simulink model "DeathOrGlory"  (R2017b)
settings: Solver=ode3  StartTime=0.0  StopTime=inf  FixedStep=0.0005  RelTol=1e-3
values from neighbouring files (symbols this model uses):
  fs = 1000    [Acquisizione_segnale_per_SVM_prova.m]    (also in training.m; warmup.m)
  interval = 192    [warmup.m]
  null_sum_finger = null_base_finger(:,1)+null_base_finger(:,2)    [matrix_h_hand_config.m]
  null_sum_thumb = null_base_thumb(:,1)+null_base_thumb(:,2)    [matrix_h_hand_config.m]
  num_act = 30    [KinematicData.m]
  pseudo_inv_h_finger = pinv(h_finger)    [matrix_h_hand_config.m]
  pseudo_inv_h_thumb = pinv(h_thumb)    [matrix_h_hand_config.m]
  pseudo_inv_h_wrist = pinv(h_wrist)    [matrix_h_hand_config.m]
  pseudo_inv_trasp_h_finger = pinv(transp(h_finger))    [matrix_h_hand_config.m]
  pseudo_inv_trasp_h_thumb = pinv(transp(h_thumb))    [matrix_h_hand_config.m]
  pseudo_inv_trasp_h_wrist = pinv(transp(h_wrist))    [matrix_h_hand_config.m]
  sM = mean(train(:,1:end-1))    [SVM_crossValidation.m]    (also in training.m; warmup.m = 0)
  sS = std(train(:,1:end-1))    [SVM_crossValidation.m]    (also in training.m; warmup.m = 0)
  Temg = 0.0005    [START_parametri_simulink.mat]    (also in matrix_h_hand_config.m)
  Ts = 0.05    [KinematicData.m]    (also in START_parametri_simulink.mat)
  w = 20    [Acquisizione_segnale_per_SVM_prova.m]    (also in warmup.m)
libraries: simulink x28, dspindex x15, dspfdesign x2, simulink_need_slupdate x2, dspmlti4 x1, dspstat3 x1, dspsrcs4 x1, simulink_extras x1
(part 2 of 2)

== system DeathOrGlory/UB Hand system1/SEND REFERENCES/dyna_send/Subsystem7 ==
  In1 : Inport
  Add : Sum  Inputs=+-
  Interval Test : simulink/Logic and Bit Operations/Interval Test  IntervalClosedRight=on  uplimit=0.1  IntervalClosedLeft=on  lowlimit=-0.1  OutDataTypeStr=boolean
  Logical Operator : Logic  Operator=NOT  AllPortsSameDT=off  OutDataTypeStr=boolean
  Unit Delay : UnitDelay  InitialCondition=zeros(30,1)  SampleTime=-1
  tag scope: changes_punch=global
  wires:
  Unit Delay/1 -> Add/2
  Add/1 -> Interval Test/1
  Interval Test/1 -> Logical Operator/1
  In1/1 -> Unit Delay/1, Add/1
  Logical Operator/1 -> [changes_punch]

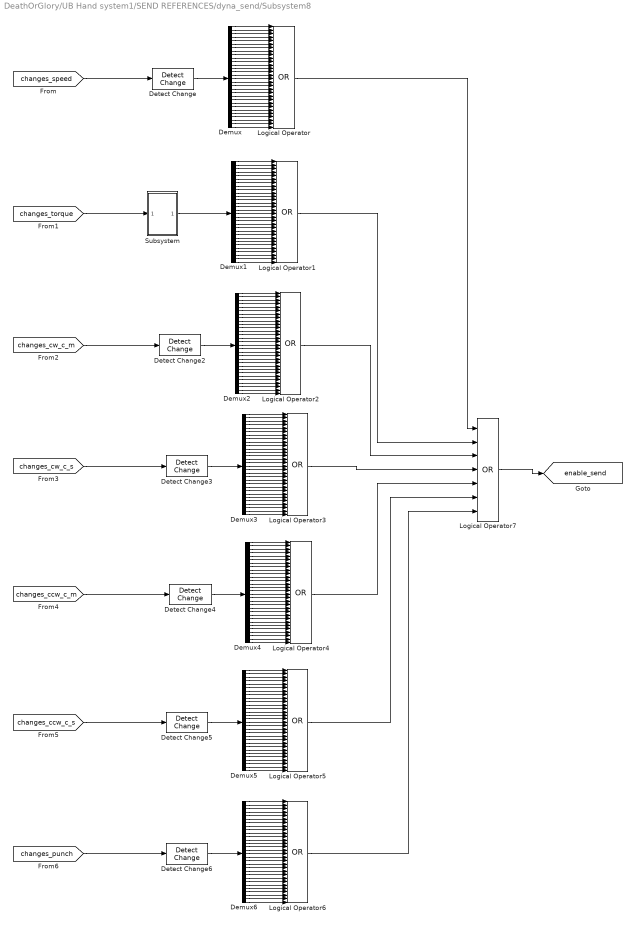
== system DeathOrGlory/UB Hand system1/SEND REFERENCES/dyna_send/Subsystem8 ==
  Demux{,1..6} (7 alike) : Demux  Outputs=30
  Detect Change{,2..6} (6 alike) : simulink/Logic and Bit Operations/Detect Change  vinit=0  InputProcessing=Columns as channels (frame based)  OutDataTypeStr=uint8
  Logical Operator{,1..6} (7 alike) : Logic  Operator=OR  Inputs=30  AllPortsSameDT=off  OutDataTypeStr=boolean
  Logical Operator7 : Logic  Operator=OR  Inputs=7  AllPortsSameDT=off  OutDataTypeStr=boolean
  Subsystem : Subsystem
  tag scope: enable_send=global
  wires:
  [changes_speed] -> Detect Change/1
  Demux/1 -> Logical Operator/1
  Demux/2 -> Logical Operator/2
  Demux/3 -> Logical Operator/3
  Demux/4 -> Logical Operator/4
  Demux/5 -> Logical Operator/5
  Demux/6 -> Logical Operator/6
  Demux/7 -> Logical Operator/7
  Demux/8 -> Logical Operator/8
  Demux/9 -> Logical Operator/9
  Demux/10 -> Logical Operator/10
  Demux/11 -> Logical Operator/11
  Demux/12 -> Logical Operator/12
  Demux/13 -> Logical Operator/13
  Demux/14 -> Logical Operator/14
  Demux/15 -> Logical Operator/15
  Demux/16 -> Logical Operator/16
  Demux/17 -> Logical Operator/17
  Demux/18 -> Logical Operator/18
  Demux/19 -> Logical Operator/19
  Demux/20 -> Logical Operator/20
  Demux/21 -> Logical Operator/21
  Demux/22 -> Logical Operator/22
  Demux/23 -> Logical Operator/23
  Demux/24 -> Logical Operator/24
  Demux/25 -> Logical Operator/25
  Demux/26 -> Logical Operator/26
  Demux/27 -> Logical Operator/27
  Demux/28 -> Logical Operator/28
  Demux/29 -> Logical Operator/29
  Demux/30 -> Logical Operator/30
  Detect Change/1 -> Demux/1
  [changes_torque] -> Subsystem/1(In1)
  Demux1/4 -> Logical Operator1/4
  Demux1/5 -> Logical Operator1/5
  Demux1/6 -> Logical Operator1/6
  Demux1/7 -> Logical Operator1/7
  Demux1/8 -> Logical Operator1/8
  Demux1/9 -> Logical Operator1/9
  Demux1/10 -> Logical Operator1/10
  Demux1/11 -> Logical Operator1/11
  Demux1/12 -> Logical Operator1/12
  Demux1/13 -> Logical Operator1/13
  Demux1/14 -> Logical Operator1/14
  Demux1/15 -> Logical Operator1/15
  Demux1/16 -> Logical Operator1/16
  Demux1/17 -> Logical Operator1/17
  Demux1/18 -> Logical Operator1/18
  Demux1/19 -> Logical Operator1/19
  Demux1/20 -> Logical Operator1/20
  Demux1/21 -> Logical Operator1/21
  Demux1/22 -> Logical Operator1/22
  Demux1/23 -> Logical Operator1/23
  Demux1/24 -> Logical Operator1/24
  Demux1/25 -> Logical Operator1/25
  Demux1/26 -> Logical Operator1/26
  Demux1/27 -> Logical Operator1/27
  Demux1/28 -> Logical Operator1/28
  Demux1/29 -> Logical Operator1/29
  Demux1/30 -> Logical Operator1/30
  Subsystem/1(Out1) -> Demux1/1
  Demux2/4 -> Logical Operator2/4
  Demux2/5 -> Logical Operator2/5
  Demux2/6 -> Logical Operator2/6
  Demux2/7 -> Logical Operator2/7
  Demux2/8 -> Logical Operator2/8
  Demux2/9 -> Logical Operator2/9
  Demux2/10 -> Logical Operator2/10
  Demux2/11 -> Logical Operator2/11
  Demux2/12 -> Logical Operator2/12
  Demux2/13 -> Logical Operator2/13
  Demux2/14 -> Logical Operator2/14
  Demux2/15 -> Logical Operator2/15
  Demux2/16 -> Logical Operator2/16
  Demux2/17 -> Logical Operator2/17
  Demux2/18 -> Logical Operator2/18
  Demux2/19 -> Logical Operator2/19
  Demux2/20 -> Logical Operator2/20
  Demux2/21 -> Logical Operator2/21
  Demux2/22 -> Logical Operator2/22
  Demux2/23 -> Logical Operator2/23
  Demux2/24 -> Logical Operator2/24
  Demux2/25 -> Logical Operator2/25
  Demux2/26 -> Logical Operator2/26
  Demux2/27 -> Logical Operator2/27
  Demux2/28 -> Logical Operator2/28
  Demux2/29 -> Logical Operator2/29
  Demux2/30 -> Logical Operator2/30
  Detect Change2/1 -> Demux2/1
  [changes_cw_c_m] -> Detect Change2/1
  Demux3/4 -> Logical Operator3/4
  Demux3/5 -> Logical Operator3/5
  Demux3/6 -> Logical Operator3/6
  Demux3/7 -> Logical Operator3/7
  Demux3/8 -> Logical Operator3/8
  Demux3/9 -> Logical Operator3/9
  Demux3/10 -> Logical Operator3/10
  Demux3/11 -> Logical Operator3/11
  Demux3/12 -> Logical Operator3/12
  Demux3/13 -> Logical Operator3/13
  Demux3/14 -> Logical Operator3/14
  Demux3/15 -> Logical Operator3/15
  Demux3/16 -> Logical Operator3/16
  Demux3/17 -> Logical Operator3/17
  Demux3/18 -> Logical Operator3/18
  Demux3/19 -> Logical Operator3/19
  Demux3/20 -> Logical Operator3/20
  Demux3/21 -> Logical Operator3/21
  Demux3/22 -> Logical Operator3/22
  Demux3/23 -> Logical Operator3/23
  Demux3/24 -> Logical Operator3/24
  Demux3/25 -> Logical Operator3/25
  Demux3/26 -> Logical Operator3/26
  Demux3/27 -> Logical Operator3/27
  Demux3/28 -> Logical Operator3/28
  Demux3/29 -> Logical Operator3/29
  Demux3/30 -> Logical Operator3/30
  Detect Change3/1 -> Demux3/1
  [changes_cw_c_s] -> Detect Change3/1
  Demux4/4 -> Logical Operator4/4
  Demux4/5 -> Logical Operator4/5
  Demux4/6 -> Logical Operator4/6
  Demux4/7 -> Logical Operator4/7
  Demux4/8 -> Logical Operator4/8
  Demux4/9 -> Logical Operator4/9
  Demux4/10 -> Logical Operator4/10
  Demux4/11 -> Logical Operator4/11
  Demux4/12 -> Logical Operator4/12
  Demux4/13 -> Logical Operator4/13
  Demux4/14 -> Logical Operator4/14
  Demux4/15 -> Logical Operator4/15
  Demux4/16 -> Logical Operator4/16
  Demux4/17 -> Logical Operator4/17
  Demux4/18 -> Logical Operator4/18
  Demux4/19 -> Logical Operator4/19
  Demux4/20 -> Logical Operator4/20
  Demux4/21 -> Logical Operator4/21
  Demux4/22 -> Logical Operator4/22
  Demux4/23 -> Logical Operator4/23
  Demux4/24 -> Logical Operator4/24
  Demux4/25 -> Logical Operator4/25
  Demux4/26 -> Logical Operator4/26
  Demux4/27 -> Logical Operator4/27
  Demux4/28 -> Logical Operator4/28
  Demux4/29 -> Logical Operator4/29
  Detect Change4/1 -> Demux4/1
  [changes_ccw_c_m] -> Detect Change4/1
  Demux5/4 -> Logical Operator5/4
  Demux5/5 -> Logical Operator5/5
  Demux5/6 -> Logical Operator5/6
  Demux5/7 -> Logical Operator5/7
  Demux5/8 -> Logical Operator5/8
  Demux5/9 -> Logical Operator5/9
  Demux5/10 -> Logical Operator5/10
  Demux5/11 -> Logical Operator5/11
  Demux5/12 -> Logical Operator5/12
  Demux5/13 -> Logical Operator5/13
  Demux5/14 -> Logical Operator5/14
  Demux5/15 -> Logical Operator5/15
  Demux5/16 -> Logical Operator5/16
  Demux5/17 -> Logical Operator5/17
  Demux5/18 -> Logical Operator5/18
  Demux5/19 -> Logical Operator5/19
  Demux5/20 -> Logical Operator5/20
  Demux5/21 -> Logical Operator5/21
  Demux5/22 -> Logical Operator5/22
  Demux5/23 -> Logical Operator5/23
  Demux5/24 -> Logical Operator5/24
  Demux5/25 -> Logical Operator5/25
  Demux5/26 -> Logical Operator5/26
  Demux5/27 -> Logical Operator5/27
  Demux5/28 -> Logical Operator5/28
  Demux5/29 -> Logical Operator5/29
  Detect Change5/1 -> Demux5/1
  [changes_ccw_c_s] -> Detect Change5/1
  Demux6/4 -> Logical Operator6/4
  Demux6/5 -> Logical Operator6/5
  Demux6/6 -> Logical Operator6/6
  Demux6/7 -> Logical Operator6/7
  Demux6/8 -> Logical Operator6/8
  Demux6/9 -> Logical Operator6/9
  Demux6/10 -> Logical Operator6/10
  Demux6/11 -> Logical Operator6/11
  Demux6/12 -> Logical Operator6/12
  Demux6/13 -> Logical Operator6/13
  Demux6/14 -> Logical Operator6/14
  Demux6/15 -> Logical Operator6/15
  Demux6/16 -> Logical Operator6/16
  Demux6/17 -> Logical Operator6/17
  Demux6/18 -> Logical Operator6/18
  Demux6/19 -> Logical Operator6/19
  Demux6/20 -> Logical Operator6/20
  Demux6/21 -> Logical Operator6/21
  Demux6/22 -> Logical Operator6/22
  Demux6/23 -> Logical Operator6/23
  Demux6/24 -> Logical Operator6/24
  Demux6/25 -> Logical Operator6/25
  Demux6/26 -> Logical Operator6/26
  Demux6/27 -> Logical Operator6/27
  Demux6/28 -> Logical Operator6/28
  Demux6/29 -> Logical Operator6/29
  Detect Change6/1 -> Demux6/1
  [changes_punch] -> Detect Change6/1
  Logical Operator1/1 -> Logical Operator7/2
  Logical Operator2/1 -> Logical Operator7/3
  Logical Operator3/1 -> Logical Operator7/4
  Logical Operator4/1 -> Logical Operator7/5
  Logical Operator5/1 -> Logical Operator7/6
  Logical Operator6/1 -> Logical Operator7/7
  Logical Operator7/1 -> [enable_send]
  Logical Operator/1 -> Logical Operator7/1
  Demux1/1 -> Logical Operator1/1
  Demux1/2 -> Logical Operator1/2
  Demux1/3 -> Logical Operator1/3
  Demux2/1 -> Logical Operator2/1
  Demux2/2 -> Logical Operator2/2
  Demux2/3 -> Logical Operator2/3
  Demux3/1 -> Logical Operator3/1
  Demux3/2 -> Logical Operator3/2
  Demux3/3 -> Logical Operator3/3
  Demux4/1 -> Logical Operator4/1
  Demux4/2 -> Logical Operator4/2
  Demux4/3 -> Logical Operator4/3
  Demux4/30 -> Logical Operator4/30
  Demux5/1 -> Logical Operator5/1
  Demux5/2 -> Logical Operator5/2
  Demux5/3 -> Logical Operator5/3
  Demux5/30 -> Logical Operator5/30
  Demux6/1 -> Logical Operator6/1
  Demux6/2 -> Logical Operator6/2
  Demux6/3 -> Logical Operator6/3
  Demux6/30 -> Logical Operator6/30

== system DeathOrGlory/UB Hand system1/TORQUE_controllo_torque2/Subsystem1/finger_convertion ==
  tau_d : Inport
  f0 : Inport  Port=2
  MATLAB Function : MATLAB Function  TreatAsAtomicUnit=on
  Matrix Multiply1 : Product  Multiplication=Matrix(*)
  Matrix Multiply3 : Product  Multiplication=Matrix(*)
  PSEUDO-INV_H_FINGER : Constant  Value=pseudo_inv_trasp_h_finger  VectorParams1D=off  SampleTime=-1
  Sum : Sum  Inputs=|++
  null_space_vetor (fk) : Constant  Value=null_sum_finger  VectorParams1D=off  SampleTime=-1
  fa : Outport
  wires:
  PSEUDO-INV_H_FINGER/1 -> Matrix Multiply1/1
  tau_d/1 -> Matrix Multiply1/2
  Matrix Multiply1/1 -> MATLAB Function/1(fm), Sum/1
  Sum/1 -> fa/1
  f0/1 -> MATLAB Function/3(f0)
  null_space_vetor (fk)/1 -> Matrix Multiply3/1, MATLAB Function/2(fk)
  Matrix Multiply3/1 -> Sum/2
  MATLAB Function/1(lambda) -> Matrix Multiply3/2

== system DeathOrGlory/UB Hand system1/TORQUE_controllo_torque2/Subsystem1/finger_convertion1 ==
  tau_d : Inport
  f0 : Inport  Port=2
  MATLAB Function : MATLAB Function  TreatAsAtomicUnit=on
  Matrix Multiply1 : Product  Multiplication=Matrix(*)
  Matrix Multiply3 : Product  Multiplication=Matrix(*)
  PSEUDO-INV_H_FINGER : Constant  Value=pseudo_inv_trasp_h_finger  VectorParams1D=off  SampleTime=-1
  Sum : Sum  Inputs=|++
  null_space_vetor (fk) : Constant  Value=null_sum_finger  VectorParams1D=off  SampleTime=-1
  fa : Outport
  wires:
  MATLAB Function/1(lambda) -> Matrix Multiply3/2
  Matrix Multiply3/1 -> Sum/2
  null_space_vetor (fk)/1 -> MATLAB Function/2(fk), Matrix Multiply3/1
  Sum/1 -> fa/1
  Matrix Multiply1/1 -> Sum/1, MATLAB Function/1(fm)
  tau_d/1 -> Matrix Multiply1/2
  PSEUDO-INV_H_FINGER/1 -> Matrix Multiply1/1
  f0/1 -> MATLAB Function/3(f0)

== system DeathOrGlory/UB Hand system1/TORQUE_controllo_torque2/Subsystem1/finger_convertion2 ==
  tau_d : Inport
  f0 : Inport  Port=2
  MATLAB Function : MATLAB Function  TreatAsAtomicUnit=on
  Matrix Multiply1 : Product  Multiplication=Matrix(*)
  Matrix Multiply3 : Product  Multiplication=Matrix(*)
  PSEUDO-INV_H_FINGER : Constant  Value=pseudo_inv_trasp_h_finger  VectorParams1D=off  SampleTime=-1
  Sum : Sum  Inputs=|++
  null_space_vetor (fk) : Constant  Value=null_sum_finger  VectorParams1D=off  SampleTime=-1
  fa : Outport
  wires:
  PSEUDO-INV_H_FINGER/1 -> Matrix Multiply1/1
  tau_d/1 -> Matrix Multiply1/2
  Matrix Multiply1/1 -> MATLAB Function/1(fm), Sum/1
  Sum/1 -> fa/1
  null_space_vetor (fk)/1 -> Matrix Multiply3/1, MATLAB Function/2(fk)
  Matrix Multiply3/1 -> Sum/2
  MATLAB Function/1(lambda) -> Matrix Multiply3/2
  f0/1 -> MATLAB Function/3(f0)

== system DeathOrGlory/UB Hand system1/TORQUE_controllo_torque2/Subsystem1/finger_convertion3 ==
  tau_d : Inport
  f0 : Inport  Port=2
  MATLAB Function : MATLAB Function  TreatAsAtomicUnit=on
  Matrix Multiply1 : Product  Multiplication=Matrix(*)
  Matrix Multiply3 : Product  Multiplication=Matrix(*)
  PSEUDO-INV_H_FINGER : Constant  Value=pseudo_inv_trasp_h_finger  VectorParams1D=off  SampleTime=-1
  Sum : Sum  Inputs=|++
  null_space_vetor (fk) : Constant  Value=null_sum_finger  VectorParams1D=off  SampleTime=-1
  fa : Outport
  wires:
  MATLAB Function/1(lambda) -> Matrix Multiply3/2
  Matrix Multiply3/1 -> Sum/2
  null_space_vetor (fk)/1 -> MATLAB Function/2(fk), Matrix Multiply3/1
  Sum/1 -> fa/1
  Matrix Multiply1/1 -> Sum/1, MATLAB Function/1(fm)
  tau_d/1 -> Matrix Multiply1/2
  PSEUDO-INV_H_FINGER/1 -> Matrix Multiply1/1
  f0/1 -> MATLAB Function/3(f0)

== system DeathOrGlory/UB Hand system1/TORQUE_controllo_torque2/Subsystem1/thumb_convertion ==
  tau_d : Inport
  f0 : Inport  Port=2
  Display : Display
  Display1 : Display
  MATLAB Function : MATLAB Function  TreatAsAtomicUnit=on
  Matrix Multiply1 : Product  Multiplication=Matrix(*)
  Matrix Multiply3 : Product  Multiplication=Matrix(*)
  PSEUDO-INV_H_FINGER : Constant  Value=pseudo_inv_trasp_h_thumb  VectorParams1D=off  SampleTime=-1
  Sum : Sum  Inputs=|++
  null_space_vetor (fk) : Constant  Value=null_sum_thumb  VectorParams1D=off  SampleTime=-1
  fa : Outport
  wires:
  null_space_vetor (fk)/1 -> Matrix Multiply3/1, MATLAB Function/2(fk)
  Sum/1 -> Display1/1, fa/1
  Matrix Multiply1/1 -> Display/1, MATLAB Function/1(fm), Sum/1
  tau_d/1 -> Matrix Multiply1/2
  PSEUDO-INV_H_FINGER/1 -> Matrix Multiply1/1
  Matrix Multiply3/1 -> Sum/2
  MATLAB Function/1(lambda) -> Matrix Multiply3/2
  f0/1 -> MATLAB Function/3(f0)

== system DeathOrGlory/UB Hand system1/TORQUE_controllo_torque2/Subsystem1/wrist_convertion ==
  tau_d : Inport
  f0 : Inport  Port=2
  Matrix Multiply1 : Product  Multiplication=Matrix(*)
  PSEUDO-INV_H_FINGER : Constant  Value=pseudo_inv_trasp_h_wrist  VectorParams1D=off  SampleTime=-1
  Sum : Sum  Inputs=|++
  fa : Outport
  wires:
  PSEUDO-INV_H_FINGER/1 -> Matrix Multiply1/1
  tau_d/1 -> Matrix Multiply1/2
  Matrix Multiply1/1 -> Sum/1
  Sum/1 -> fa/1
  f0/1 -> Sum/2

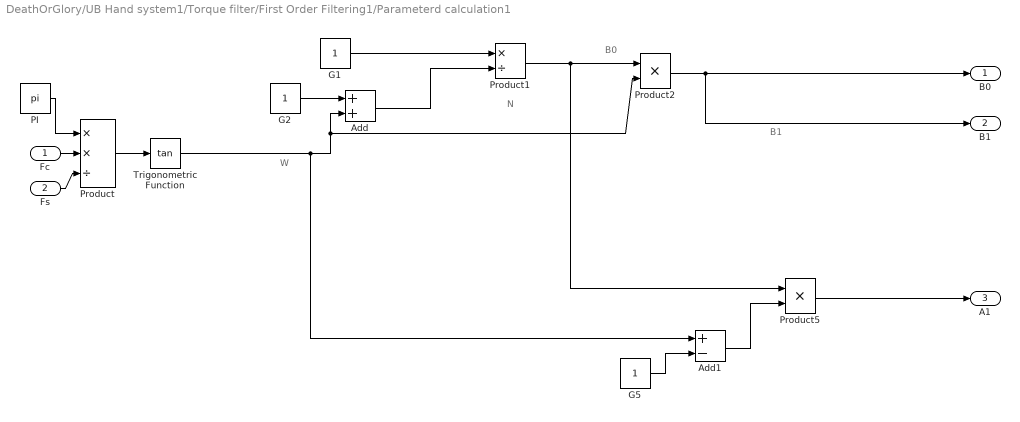
== system DeathOrGlory/UB Hand system1/Torque filter/First Order Filtering1/Parameterd calculation1 ==
  note: N
  note: W
  note: B0
  note: B1
  Fc : Inport
  Fs : Inport  Port=2
  Add : Sum
  Add1 : Sum  Inputs=+-
  G1 : Constant  SampleTime=-1
  G2 : Constant  SampleTime=-1
  G5 : Constant  SampleTime=-1
  PI : Constant  Value=pi  SampleTime=-1
  Product : Product  Inputs=**/  RndMeth=Zero
  Product1 : Product  Inputs=*/  RndMeth=Zero
  Product2 : Product  Inputs=**  RndMeth=Zero
  Product5 : Product  Inputs=**  RndMeth=Zero
  Trigonometric Function : Trigonometry  Operator=tan
  B0 : Outport
  B1 : Outport  Port=2
  A1 : Outport  Port=3
  wires:
  Product2/1 -> B1/1, B0/1
  Product1/1 -> Product2/1, Product5/1
  Add/1 -> Product1/2
  G1/1 -> Product1/1
  G2/1 -> Add/1
  Trigonometric Function/1 -> Product2/2, Add/2, Add1/1
  Product/1 -> Trigonometric Function/1
  PI/1 -> Product/1
  Fc/1 -> Product/2
  Fs/1 -> Product/3
  G5/1 -> Add1/2
  Add1/1 -> Product5/2
  Product5/1 -> A1/1

== system DeathOrGlory/UB Hand system1/SEND REFERENCES/dyna_send/Subsystem8/Subsystem ==
  In1 : Inport
  Add : Sum  Inputs=+-
  Interval Test : simulink/Logic and Bit Operations/Interval Test  IntervalClosedRight=on  uplimit=0.1  IntervalClosedLeft=on  lowlimit=-0.1  OutDataTypeStr=boolean
  Logical Operator : Logic  Operator=NOT  AllPortsSameDT=off  OutDataTypeStr=boolean
  Unit Delay : UnitDelay  SampleTime=-1
  Out1 : Outport
  wires:
  Unit Delay/1 -> Add/2
  Add/1 -> Interval Test/1
  Interval Test/1 -> Logical Operator/1
  In1/1 -> Add/1, Unit Delay/1
  Logical Operator/1 -> Out1/1

== matlab function DeathOrGlory/UB Hand system1/SEND REFERENCES/Position_Estimation/MATLAB Function1 ==
  data: mot_ref_in input; mot_ref_out output
function mot_ref_out  = fcn(mot_ref_in)
%#codegen
mot_ref_supp=zeros(30,1);
num_mot_thumb=[13 14 10 12 11];
sign_thumb=  [-1 1 1 1 -1];
num_mot_index=[8 9 7 5 6];
sign_index=[ 1 -1 -1 -1 1];
num_mot_middle=[2 4 3 27 28];
sign_middle=[ 1 1 -1 1 -1];
num_mot_ring=[24 26 25 21 23];
sign_ring=[ -1 -1 1 1 1];
num_mot_little=[20 22 19 17 18];
sign_little=[-1 -1 1 1 -1];
num_mot_wrist=[15 16 1 30];
sign_wrist=[-1 1 -1 -1];
free_mot= 29;
sign_free= -1;
num_mot= [num_mot_thumb num_mot_index num_mot_middle num_mot_ring num_mot_little num_mot_wrist free_mot];
sign= [sign_thumb sign_index sign_middle sign_ring sign_little sign_wrist sign_free];

for i=1:30

        if sign(i)== 1 
            
                mot_ref_supp(i)=-mot_ref_in(i);

           
        end
        
         if sign(i)== -1
             
                mot_ref_supp(i)=mot_ref_in(i);
            
         end
end



mot_ref_supp(30)=0;
mot_ref_out = mot_ref_supp;

== matlab function DeathOrGlory/EMG system/MATLAB Function ==
  data: u input; ch1 output; ch2 output; ch3 output; ch4 output; ch5 output; ch6 output; ch7 output; ch8 output
function [ch1,ch2,ch3,ch4,ch5,ch6,ch7,ch8] = fcn(u)
% [ch1,ch2,ch3,ch4,ch5,ch6,ch7,ch8] = fcn(u)

    a=true;
    
    nbytes=0;
    
    data=zeros(22,1);

    coder.extrinsic('serial', 'fopen','fprintf','get','instrfind','display');
    
    persistent s
    persistent c1
    persistent c2
    persistent c3
    persistent c4
    persistent c5
    persistent c6
    persistent c7
    persistent c8
    
    if isempty(s)

        disp('sono dentro isempty');
        
        a=isempty(instrfind);
        if a==0
            fclose(instrfind);
        end
        
        s = serial('COM40');

        set(s,'InputBufferSize',10000000);
        fopen(s);
        
%         pause on;
%         
%         disp('pausa... ...');
%         
%         pause(30);

        fprintf(s,'=');
        
        c1=0; c2=0; c3=0; c4=0;
        c5=0; c6=0; c7=0; c8=0;
    end
    
    
    %disp('reading...');
    byte1=0; byte2=0; 
    byte3=0; byte4=0; 
    byte5=0; byte6=0;
    byte7=0; byte8=0;
    byte9=0; byte10=0;
    byte11=0; byte12=0;
    byte13=0; byte14=0;
    byte15=0; byte16=0;
    byte17=0; byte18=0;
    byte19=0; byte20=0;
    byte21=0; byte22=0;
    
    nbytes=get(s,'BytesAvailable');
    %display(nbytes)
    
    if u < 1 %&& nbytes>=22

         data = fread(s,22,'uint8');
         %data(1)=(typecast(uint8(data(1)),'int8'));

        if data(1) == 32            
            
            byte4=double(data(4));
            byte5=double(typecast(uint8(data(5)),'int8'));
            byte6=double(data(6));
            byte7=double(typecast(uint8(data(7)),'int8'));
            byte8=double(data(8));
            byte9=double(typecast(uint8(data(9)),'int8'));
            byte10=double(data(10));
            byte11=double(typecast(uint8(data(11)),'int8'));
            byte12=double(data(12));
            byte13=double(typecast(uint8(data(13)),'int8'));
            byte14=double(data(14));
            byte15=double(typecast(uint8(data(15)),'int8'));
            byte16=double(data(16));
            byte17=double(typecast(uint8(data(17)),'int8'));
            byte18=double(data(18));
            byte19=double(typecast(uint8(data(19)),'int8'));
            byte20=double(data(20));
            byte21=double(data(21));

            if byte20==0 && byte21==0
                c1=byte4+byte5*256;
                c2=byte6+byte7*256;
                c3=byte8+byte9*256;
                c4=byte10+byte11*256;
                c5=byte12+byte13*256;
                c6=byte14+byte15*256;
                c7=byte16+byte17*256;
                c8=byte18+byte19*256;
            end
        end
    end

ch1 = c1(1);
ch2 = c2(1);
ch3 = c3(1);
ch4 = c4(1);
ch5 = c5(1);
ch6 = c6(1);
ch7 = c7(1);
ch8 = c8(1);

if u>0
    fprintf(s,':');
end

== matlab function DeathOrGlory/UB Hand system1/SEND REFERENCES/Joints2Motor/operative_mode//calibration_mode/MATLAB Function2 ==
  data: mot_ref_in input; mot_ref_out output
function mot_ref_out  = fcn(mot_ref_in)
%#codegen
mot_ref_supp=zeros(30,1);
num_mot_thumb=[13 14 10 12 11];
sign_thumb=  [-1 1 1 1 -1];
num_mot_index=[8 9 7 5 6];
sign_index=[ 1 -1 -1 -1 1];
num_mot_middle=[2 4 3 27 28];
sign_middle=[ 1 1 -1 1 -1];
num_mot_ring=[24 26 25 21 23];
sign_ring=[ -1 -1 1 1 1];
num_mot_little=[20 22 19 17 18];
sign_little=[-1 -1 1 1 -1];
num_mot_wrist=[15 16 1 30];
sign_wrist=[-1 1 -1 -1];
free_mot= 29;
sign_free= -1;
num_mot= [num_mot_thumb num_mot_index num_mot_middle num_mot_ring num_mot_little num_mot_wrist free_mot];
sign= [sign_thumb sign_index sign_middle sign_ring sign_little sign_wrist sign_free];

for i=1:30

        if sign(i)== 1 
            
                mot_ref_supp(i)=mot_ref_in(i);

           
        end
        
         if sign(i)== -1
             
                mot_ref_supp(i)=280-mot_ref_in(i);
            
         end
end



mot_ref_supp(30)=0;
mot_ref_out = mot_ref_supp;

== matlab function DeathOrGlory/UB Hand system1/SEND REFERENCES/MATLAB Function1 ==
  data: torque_in input; free_lx input; free_rx input; torque_out output; activate_wrist input
function torque_out  = fcn(torque_in,free_lx,free_rx,activate_wrist)
torque_supp=zeros(30,1);
num_mot_thumb=[13 14 10 12 11];

num_mot_index=[8 9 7 5 6];

num_mot_middle=[2 4 3 27 28];

num_mot_ring=[24 26 25 21 23];

num_mot_little=[20 22 19 17 18];

num_mot_wrist=[15 16 1 30];

free_mot= 29;

num_mot= [num_mot_thumb num_mot_index num_mot_middle num_mot_ring num_mot_little num_mot_wrist free_mot];


for i=1:30

            if  num_mot(i)<17
                if free_lx==1
               torque_supp(i)=0;
            else 
                 torque_supp(i)=torque_in(i);
                end
            else
            
            if num_mot(i)>16
                if free_rx==1
               torque_supp(i)=0;
            else
                torque_supp(i)=torque_in(i);
                end
            end
            end
        
      
end

   if activate_wrist==1
               torque_supp(26:29)=torque_in(26:29);
   end

torque_supp(30)=0;
torque_out = torque_supp;

== matlab function DeathOrGlory/Estrazione feature/MATLAB Function ==
  data: d1 input; y output; d2 input; d3 input; d4 input
function y = marginals(d1, d2, d3, d4)

%calcoliamo i marginals per ogni livello di decomposizione
m1=sum(abs(d1));
m2=sum(abs(d2));
m3=sum(abs(d3));
m4=sum(abs(d4));
h=1;

%generiamo il vettore che li contiene tutti per ogni canale
M=zeros(1,32);
for i=1:1:8
    M(1,h:h+3)=[m1(i), m2(i), m3(i), m4(i)];
    h=h+4;
end
y = M';

== matlab function DeathOrGlory/Estrazione feature/MATLAB Function1 ==
  data: u input; y output; sM input; sS input
%normalizza i valori per poi passarli al classificatore
function y = norm(u, sM, sS)
u = (u - sM) ./ sS;
y = u;

== matlab function DeathOrGlory/Estrazione feature/online_SVM_gesture_classification ==
  data: M input; model parameter; prediction output
function prediction = fcn(M, model)

%importo comandi non supportati dal matlab function block di simulink
coder.extrinsic('sparse','display','classification');

complete=M';

%necessario inizializzare l'output altrimenti dà errore
prediction=0;

%CHIAMO LA FUNZIONE PER ESEGUIRE LA CLASSIFICAZIONE (è necessario fare così
%perchè simulink non supporta le matrici sparse)
%lab_1= una label random
%complete= campione multidimensionale attuale da classificare
%model= modello della svm calcolato in svm_train.m e importato nella
%matlab function come "parametro"
lab_1=1;
output = classification(lab_1, complete, model);

%ritorno il risutato della classificazione
prediction = output;

== matlab function DeathOrGlory/Estrazione feature/MATLAB Function2 ==
  data: u input; y output
function y = moda(u)

uscita=0;
coder.extrinsic('mode');

uscita=mode(u);
y=uscita(1,1);

== matlab function DeathOrGlory/Homing/MATLAB Function ==
  data: u input; y output; out input
function y = fcn(u, out)
if u==7
    y=out;
else
    y = u;
end

== matlab function DeathOrGlory/UB Hand system1/SEND REFERENCES/Joints2Motor/MATLAB Function1 ==
  data: mot_ref_in input; mot_ref_out output
function mot_ref_out  = fcn(mot_ref_in)
%#codegen
mot_ref_supp=zeros(30,1);
num_mot_thumb=[13 14 10 12 11];
sign_thumb=  [-1 1 1 1 -1];
num_mot_index=[8 9 7 5 6];
sign_index=[ 1 -1 -1 -1 1];
num_mot_middle=[2 4 3 27 28];
sign_middle=[ 1 1 -1 1 -1];
num_mot_ring=[24 26 25 21 23];
sign_ring=[ -1 -1 1 1 1];
num_mot_little=[20 22 19 17 18];
sign_little=[-1 -1 1 1 -1];
num_mot_wrist=[15 16 1 30];
sign_wrist=[-1 1 -1 -1];
free_mot= 29;
sign_free= -1;
num_mot= [num_mot_thumb num_mot_index num_mot_middle num_mot_ring num_mot_little num_mot_wrist free_mot];
sign= [sign_thumb sign_index sign_middle sign_ring sign_little sign_wrist sign_free];

for i=1:30

        if sign(i)== 1 
            
                mot_ref_supp(i)=mot_ref_in(i);

           
        end
        
         if sign(i)== -1
             
                mot_ref_supp(i)=-mot_ref_in(i);
            
         end
end



mot_ref_supp(30)=0;
mot_ref_out = mot_ref_supp;

== matlab function DeathOrGlory/UB Hand system1/TORQUE_controllo_torque2/Subsystem1/finger_convertion/MATLAB Function ==
  data: fm input; lambda output; fk input; f0 input
function lambda = fcn(fm,fk,f0)

lambda_temp=zeros(5,1);

for i=1:5
    lambda_temp(i)=(f0(i)-fm(i))/fk(i);
end

lambda = max(lambda_temp);

== matlab function DeathOrGlory/UB Hand system1/TORQUE_controllo_torque2/Subsystem1/finger_convertion1/MATLAB Function ==
  data: fm input; lambda output; fk input; f0 input
function lambda = fcn(fm,fk,f0)

lambda_temp=zeros(5,1);

for i=1:5
    lambda_temp(i)=(f0(i)-fm(i))/fk(i);
end

lambda = max(lambda_temp);

== matlab function DeathOrGlory/UB Hand system1/TORQUE_controllo_torque2/Subsystem1/finger_convertion2/MATLAB Function ==
  data: fm input; lambda output; fk input; f0 input
function lambda = fcn(fm,fk,f0)

lambda_temp=zeros(5,1);

for i=1:5
    lambda_temp(i)=(f0(i)-fm(i))/fk(i);
end

lambda = max(lambda_temp);

== matlab function DeathOrGlory/UB Hand system1/TORQUE_controllo_torque2/Subsystem1/finger_convertion3/MATLAB Function ==
  data: fm input; lambda output; fk input; f0 input
function lambda = fcn(fm,fk,f0)

lambda_temp=zeros(5,1);

for i=1:5
    lambda_temp(i)=(f0(i)-fm(i))/fk(i);
end

lambda = max(lambda_temp);

== matlab function DeathOrGlory/UB Hand system1/TORQUE_controllo_torque2/Subsystem1/thumb_convertion/MATLAB Function ==
  data: fm input; lambda output; fk input; f0 input
function lambda = fcn(fm,fk,f0)

lambda_temp=zeros(5,1);

for i=1:5
    lambda_temp(i)=(f0(i)-fm(i))/fk(i);
end

lambda = max(lambda_temp);
